simulink model "obs_ard_1912_final"  (R2021a)
settings: Solver=ode4  StartTime=0.0  StopTime=inf  FixedStep=0.001  RelTol=1e-3  EnableMultiTasking=on
values from neighbouring files (symbols this model uses):
  A = [-Ra/La -Kg/(Kt*La) ... (first row only)    [observador.m]    (also in observador_arduino.m)
  B = [1/La ; 0]    [observador_arduino.m]
  C = [0 1]    [observador_arduino.m]
  K_prime = [Kt_control_1 Kt_control_2]    [observador_arduino.m]
  ki = double(solve(coeffs_det_A_r(end-3)==pol_caract(4), ki))    [observador_arduino.m]
  L = place(A', C', desired_poles)'    [observador_arduino.m]
libraries: arduinolib x2
settings Model: SILPILModeSetting=veronly  ExtModeTrigDuration=2  Creator=carol  LastModifiedBy=carol
settings OptimizationCC: EnhancedBackFolding=on  PassReuseOutputArgsAs=Individual arguments  ZeroExternalMemoryAtStartup=off  ZeroInternalMemoryAtStartup=off  MaxStackSize=64  OptimizeBlockOrder=speed  DifferentSizesBufferReuse=on  OptimizationCustomize=off  EfficientTunableParamExpr=on
settings DebuggingCC: ParameterTunabilityLossMsg=error
settings HardwareCC: ProdBitPerPointer=32  ProdBitPerSizeT=32  ProdBitPerPtrDiffT=32  ProdLargestAtomicInteger=Long  ProdLargestAtomicFloat=Double  ProdWordSize=32  ProdHWDeviceType=ARM Compatible->ARM Cortex  UseEmbeddedCoderFeatures=off  UseSimulinkCoderFeatures=off
settings SFSimCC: MATLABDynamicMemAlloc=off
settings RTWCC: SystemTargetFile=ert.tlc  HardwareBoard=Arduino Due  TemplateMakefile=ert_default_tmf  Toolchain=Arduino ARM  BuildConfiguration=Faster Runs
settings CodeAppCC: ForceParamTrailComments=on  IgnoreCustomStorageClasses=off  OperatorAnnotations=on  SimulinkDataObjDesc=on  SFDataObjDesc=on  InsertBlockDesc=on
settings ERTTargetCC: SupportContinuousTime=on  SupportNonInlinedSFcns=on  SupportVariableSizeSignals=on  ExtModeTransport=3  ExtModeStaticAlloc=on  ExtModeStaticAllocSize=24576  ExtModeMexFile=ext_xcp  ExtModeIntrfLevel=Level2 - Open

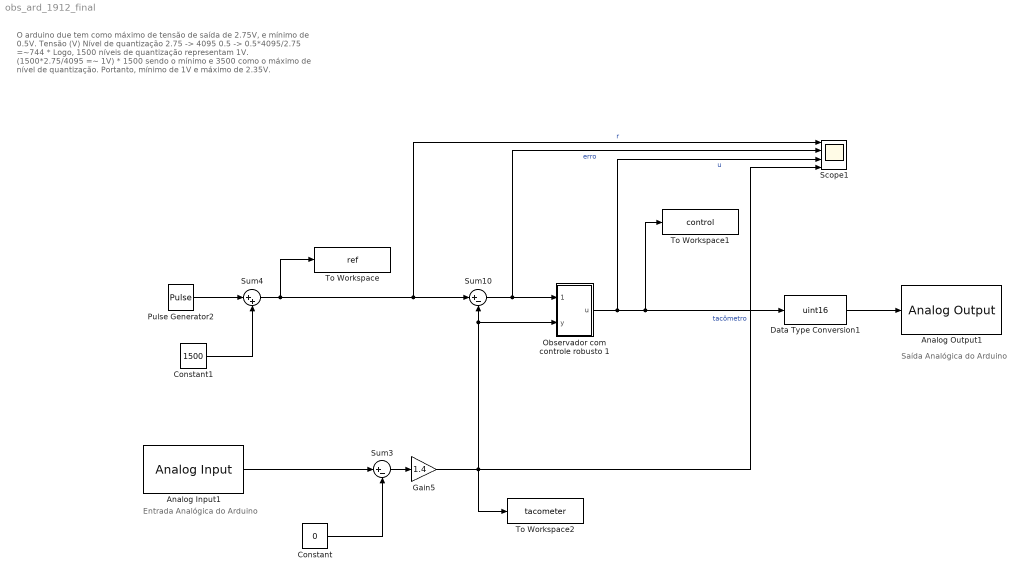
== system obs_ard_1912_final ==
  note: O arduino due tem como máximo de tensão de saída de 2.75V, e mínimo de 0.5V.
      |
      | Tensão (V) Nível de quantização
      | 2.75 -> 4095
      | 0.5 -> 0.5*4095/2.75 =~744
      |
      | * Logo, 1500 níveis de quantização
      | representam 1V.
      | (1500*2.75/4095 =~ 1V)
      |
      | * 1500 sendo o mínimo e 3500 como o máximo de nível de quantização. Portanto,
      | mínimo de 1V e máximo de 2.35V.
  note: Saída Analógica do Arduino
  note: Entrada Analógica do Arduino
  Analog Input1 : arduinolib/Analog Input  pinNumber=1  ReadResultsOnly=off  ConversionTriggerSource=Software  ExternalTriggerType=uint32( 0 )  OutputDataType=uint16  EnableConversionCompleteNotify=off  EnableOuputStatus=off  SampleTime=-1  blockPlatform=arduino
  Analog Output1 : arduinolib/Analog Output  DACpin=DAC0  blockPlatform=arduino
      settings: SourceProductBaseCode=ARDUINO
  Constant : Constant  Value=0
  Constant1 : Constant  Value=1500
  Data Type Conversion1 : DataTypeConversion  OutDataTypeStr=uint16
  Gain5 : Gain  Gain=1.4
  Observador com controle robusto 1 : Subsystem
  Pulse Generator2 : DiscretePulseGenerator  PulseType=Time based  Amplitude=2000  Period=3  PulseWidth=50
  Scope1 : Scope  NumInputPorts=4
  Sum10 : Sum  Inputs=|+-
  Sum3 : Sum  Inputs=|+-
  Sum4 : Sum  Inputs=|++
  To Workspace : ToWorkspace  VariableName=ref  SaveFormat=Structure With Time  SampleTime=-1
  To Workspace1 : ToWorkspace  VariableName=control  SaveFormat=Structure With Time  SampleTime=-1
  To Workspace2 : ToWorkspace  VariableName=tacometer  SaveFormat=Structure With Time  SampleTime=-1
  wires:
  Data Type Conversion1/1 -> Analog Output1/1
  Constant/1 -> Sum3/2
  Pulse Generator2/1 -> Sum4/1
  Gain5/1 -> Observador com controle robusto 1/2(y), Sum10/2, Scope1/4, To Workspace2/1  "tacômetro"
  Sum3/1 -> Gain5/1
  Analog Input1/1 -> Sum3/1
  Sum4/1 -> Scope1/1, Sum10/1, To Workspace/1  "r"
  Observador com controle robusto 1/1(u) -> Scope1/3, Data Type Conversion1/1, To Workspace1/1  "u"
  Sum10/1 -> Observador com controle robusto 1/1(erro), Scope1/2  "erro"
  Constant1/1 -> Sum4/2

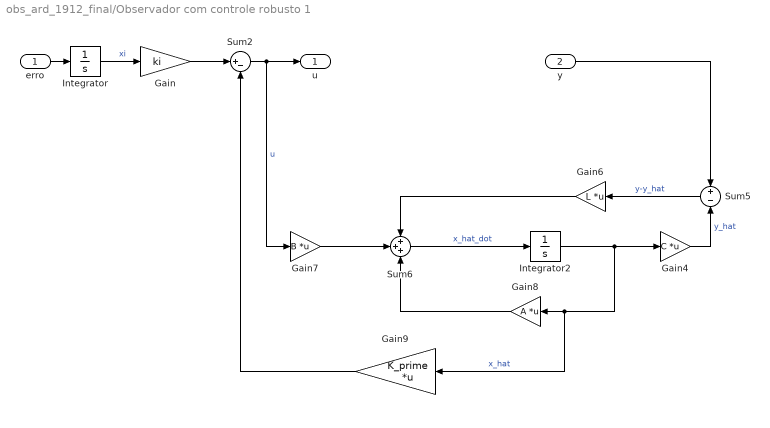
== system obs_ard_1912_final/Observador com controle robusto 1 ==
  erro : Inport
  y : Inport  Port=2
  Gain : Gain  Gain=ki
  Gain4 : Gain  Gain=C  Multiplication=Matrix(K*u)
  Gain6 : Gain  Gain=L  Multiplication=Matrix(K*u)
  Gain7 : Gain  Gain=B  Multiplication=Matrix(K*u)
  Gain8 : Gain  Gain=A  Multiplication=Matrix(K*u)
  Gain9 : Gain  Gain=K_prime  Multiplication=Matrix(K*u)
  Integrator : Integrator
  Integrator2 : Integrator  InitialCondition=6
  Sum2 : Sum  Inputs=|+-
  Sum5 : Sum  Inputs=+|-
  Sum6 : Sum  Inputs=+++
  u : Outport
  wires:
  y/1 -> Sum5/1
  Integrator2/1 -> Gain9/1, Gain8/1, Gain4/1  "x_hat"
  Integrator/1 -> Gain/1  "xi"
  Gain4/1 -> Sum5/2  "y_hat"
  Gain/1 -> Sum2/1
  Sum5/1 -> Gain6/1  "y-y_hat"
  Gain6/1 -> Sum6/1
  Gain9/1 -> Sum2/2
  Gain7/1 -> Sum6/2
  Gain8/1 -> Sum6/3
  Sum6/1 -> Integrator2/1  "x_hat_dot"
  Sum2/1 -> u/1, Gain7/1  "u"
  erro/1 -> Integrator/1
